simulink model "controllo_disco_rigido_disturbi"  (R2019b)
settings: Solver=VariableStepAuto  StartTime=0.0  StopTime=5  FixedStep=0.01  RelTol=1e-3
values from neighbouring files (symbols this model uses):
  b = 0.002    [controllo_disco_rigido.m]    (also in controllo_disco_rigido_baseWS.mat; controllo_disco_rigido_script.m; init_controllo_disco_rigido.m)
  J = 0.001    [controllo_disco_rigido.m]    (also in controllo_disco_rigido_baseWS.mat; controllo_disco_rigido_script.m; init_controllo_disco_rigido.m)
  R1 = 100    [controllo_disco_rigido.m]    (also in controllo_disco_rigido_script.m = 10^(round((((Ed)+20*wd(end))/20)-1))/gsys(3))
  R2_pole = [-500]    [controllo_disco_rigido_script.m]
  R2_zero = [-2]    [controllo_disco_rigido_script.m]
  y0 = 300    [controllo_disco_rigido.m]    (also in controllo_disco_rigido_script.m)
settings Model: Creator=Utente  LastModifiedBy=Utente
settings DataIOCC: SaveOutput=off  SignalLogging=off  DSMLogging=off  ReturnWorkspaceOutputsName=MdlCL

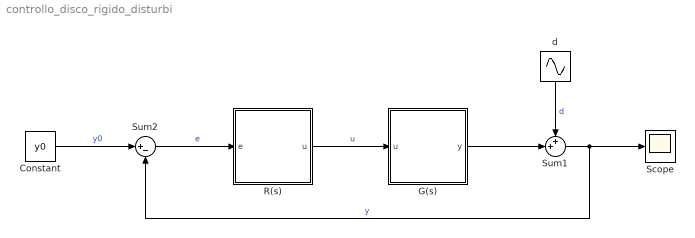
== system controllo_disco_rigido_disturbi ==
  Constant : Constant  Value=y0
  G(s) : Subsystem
  R(s) : Subsystem
  Scope : Scope
  Sum1 : Sum  Inputs=++|
  Sum2 : Sum  Inputs=|+-
  d : Sin  Frequency=[2.75]  SampleTime=0
  wires:
  R(s)/1(u) -> G(s)/1(u)  "u"
  Sum1/1 -> Scope/1, Sum2/2  "y"
  Constant/1 -> Sum2/1  "y0"
  d/1 -> Sum1/1  "d"
  G(s)/1(y) -> Sum1/2
  Sum2/1 -> R(s)/1(e)  "e"

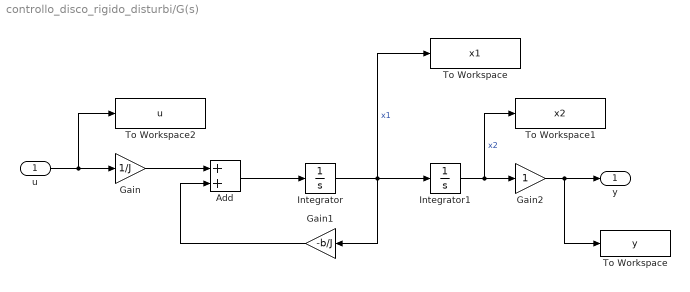
== system controllo_disco_rigido_disturbi/G(s) ==
  u : Inport
  " To Workspace" : ToWorkspace  VariableName=y  SampleTime=-1
  Add : Sum
  Gain : Gain  Gain=1/J
  Gain1 : Gain  Gain=-b/J
  Gain2 : Gain
  Integrator : Integrator
  Integrator1 : Integrator
  To Workspace : ToWorkspace  VariableName=x1  SampleTime=-1
  To Workspace1 : ToWorkspace  VariableName=x2  SampleTime=-1
  To Workspace2 : ToWorkspace  VariableName=u  SampleTime=-1
  y : Outport
  wires:
  Integrator/1 -> To Workspace/1, Gain1/1, Integrator1/1  "x1"
  u/1 -> Gain/1, To Workspace2/1
  Add/1 -> Integrator/1
  Gain/1 -> Add/1
  Gain1/1 -> Add/2
  Integrator1/1 -> Gain2/1, To Workspace1/1  "x2"
  Gain2/1 -> " To Workspace"/1, y/1

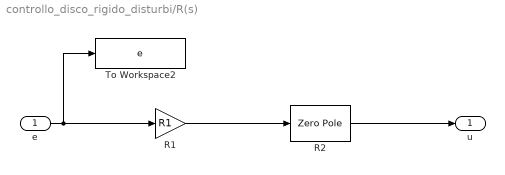
== system controllo_disco_rigido_disturbi/R(s) ==
  e : Inport
  R1 : Gain  Gain=R1
  R2 : ZeroPole  Zeros=R2_zero  Poles=R2_pole
  To Workspace2 : ToWorkspace  VariableName=e  SampleTime=-1
  u : Outport
  wires:
  R2/1 -> u/1
  R1/1 -> R2/1
  e/1 -> To Workspace2/1, R1/1
